simulink model "controller_compare"  (R2023a)
settings: Solver=VariableStepAuto  StartTime=0.0  StopTime=10.0  RelTol=1e-3
model workspace (MAT data in the model file):
  xinit = 1
settings Model: Creator=belov  LastModifiedBy=belov

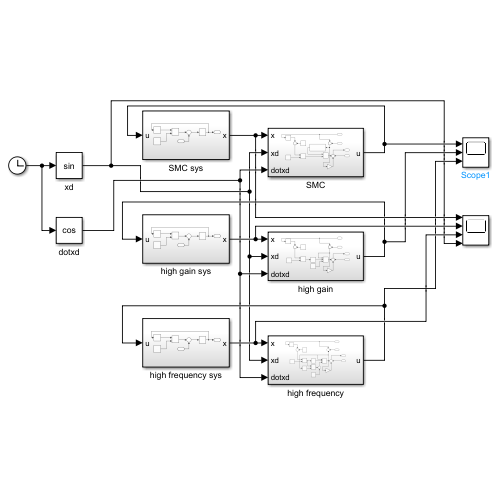
[thumbnail: Simulink's stored preview of the top-level diagram]
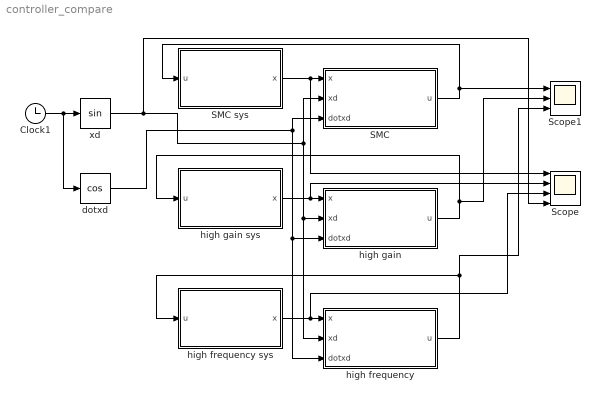
== system controller_compare ==
  Clock1 : Clock
  SMC : Subsystem
  SMC sys : Subsystem
  Scope : Scope  NumInputPorts=4
  Scope1 : Scope  NumInputPorts=3
  dotxd : Trigonometry  Operator=cos
  high frequency : Subsystem
  high frequency sys : Subsystem
  high gain : Subsystem
  high gain sys : Subsystem
  xd : Trigonometry
  wires:
  high frequency sys/1(x) -> Scope/3, high frequency/1(x)
  high gain sys/1(x) -> Scope/2, high gain/1(x)
  SMC sys/1(x) -> Scope/1, SMC/1(x)
  SMC/1(u) -> Scope1/1, SMC sys/1(u)
  high gain/1(u) -> Scope1/2, high gain sys/1(u)
  high frequency/1(u) -> Scope1/3, high frequency sys/1(u)
  xd/1 -> Scope/4, high frequency/2(xd), high gain/2(xd), SMC/2(xd)
  dotxd/1 -> SMC/3(dotxd), high frequency/3(dotxd), high gain/3(dotxd)
  Clock1/1 -> dotxd/1, xd/1

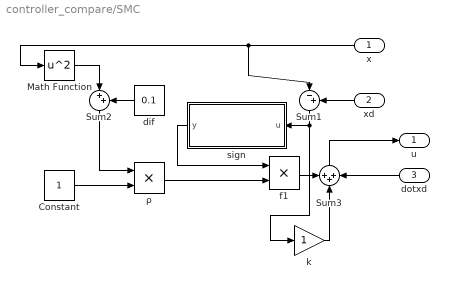
== system controller_compare/SMC ==
  x : Inport
  xd : Inport  Port=2
  dotxd : Inport  Port=3
  Constant : Constant
  Math Function : Math  Operator=square
  Sum1 : Sum  Inputs=|-+
  Sum2 : Sum  Inputs=|++
  Sum3 : Sum  Inputs=+++
  dif : Constant  Value=0.1
  f1 : Product  Inputs=**
  k : Gain
  sign : MATLAB Function  TreatAsAtomicUnit=on
  ρ : Product  Inputs=**
  u : Outport
  wires:
  Math Function/1 -> Sum2/1
  dotxd/1 -> Sum3/3
  xd/1 -> Sum1/2
  x/1 -> Sum1/1, Math Function/1
  Sum1/1 -> k/1, sign/1(u)
  Constant/1 -> ρ/2
  k/1 -> Sum3/2
  Sum2/1 -> ρ/1
  f1/1 -> Sum3/1
  dif/1 -> Sum2/2
  Sum3/1 -> u/1
  ρ/1 -> f1/2
  sign/1(y) -> f1/1

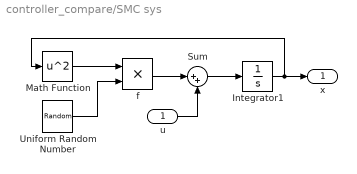
== system controller_compare/SMC sys ==
  u : Inport
  Integrator1 : Integrator  InitialCondition=1
  Math Function : Math  Operator=square
  Sum : Sum  Inputs=|++
  Uniform Random Number : UniformRandomNumber  SampleTime=0.1
  f : Product  Inputs=**
  x : Outport
  wires:
  Math Function/1 -> f/1
  f/1 -> Sum/1
  u/1 -> Sum/2
  Uniform Random Number/1 -> f/2
  Integrator1/1 -> Math Function/1, x/1
  Sum/1 -> Integrator1/1

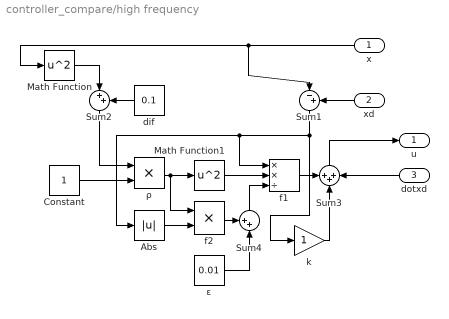
== system controller_compare/high frequency ==
  x : Inport
  xd : Inport  Port=2
  dotxd : Inport  Port=3
  Abs : Abs  SaturateOnIntegerOverflow=off
  Constant : Constant
  Math Function : Math  Operator=square
  Math Function1 : Math  Operator=square
  Sum1 : Sum  Inputs=|-+
  Sum2 : Sum  Inputs=|++
  Sum3 : Sum  Inputs=+++
  Sum4 : Sum  Inputs=++|
  dif : Constant  Value=0.1
  f1 : Product  Inputs=**/
  f2 : Product  Inputs=**
  k : Gain
  ε : Constant  Value=0.01
  ρ : Product  Inputs=**
  u : Outport
  wires:
  Math Function/1 -> Sum2/1
  dotxd/1 -> Sum3/3
  xd/1 -> Sum1/2
  x/1 -> Sum1/1, Math Function/1
  Sum1/1 -> k/1, f1/1, Abs/1
  Constant/1 -> ρ/2
  ρ/1 -> f2/1, Math Function1/1
  k/1 -> Sum3/2
  Sum2/1 -> ρ/1
  f1/1 -> Sum3/1
  dif/1 -> Sum2/2
  Sum3/1 -> u/1
  Math Function1/1 -> f1/2
  Abs/1 -> f2/2
  Sum4/1 -> f1/3
  f2/1 -> Sum4/1
  ε/1 -> Sum4/2

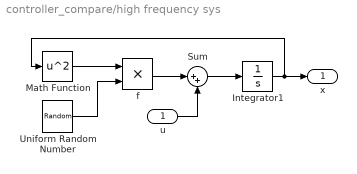
== system controller_compare/high frequency sys ==
  u : Inport
  Integrator1 : Integrator  InitialCondition=1
  Math Function : Math  Operator=square
  Sum : Sum  Inputs=|++
  Uniform Random Number : UniformRandomNumber  SampleTime=0.1
  f : Product  Inputs=**
  x : Outport
  wires:
  Math Function/1 -> f/1
  f/1 -> Sum/1
  u/1 -> Sum/2
  Uniform Random Number/1 -> f/2
  Integrator1/1 -> Math Function/1, x/1
  Sum/1 -> Integrator1/1

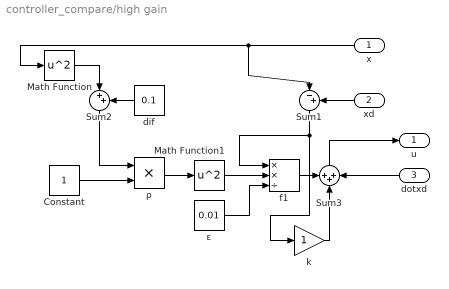
== system controller_compare/high gain ==
  x : Inport
  xd : Inport  Port=2
  dotxd : Inport  Port=3
  Constant : Constant
  Math Function : Math  Operator=square
  Math Function1 : Math  Operator=square
  Sum1 : Sum  Inputs=|-+
  Sum2 : Sum  Inputs=|++
  Sum3 : Sum  Inputs=+++
  dif : Constant  Value=0.1
  f1 : Product  Inputs=**/
  k : Gain
  ε : Constant  Value=0.01
  ρ : Product  Inputs=**
  u : Outport
  wires:
  ε/1 -> f1/3
  Math Function1/1 -> f1/2
  Sum3/1 -> u/1
  dif/1 -> Sum2/2
  f1/1 -> Sum3/1
  Sum2/1 -> ρ/1
  k/1 -> Sum3/2
  ρ/1 -> Math Function1/1
  Constant/1 -> ρ/2
  Sum1/1 -> f1/1, k/1
  x/1 -> Math Function/1, Sum1/1
  xd/1 -> Sum1/2
  dotxd/1 -> Sum3/3
  Math Function/1 -> Sum2/1

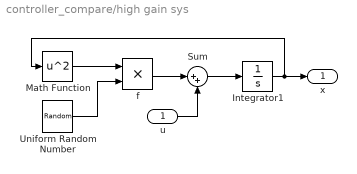
== system controller_compare/high gain sys ==
  u : Inport
  Integrator1 : Integrator  InitialCondition=1
  Math Function : Math  Operator=square
  Sum : Sum  Inputs=|++
  Uniform Random Number : UniformRandomNumber  SampleTime=0.1
  f : Product  Inputs=**
  x : Outport
  wires:
  Sum/1 -> Integrator1/1
  Integrator1/1 -> x/1, Math Function/1
  Uniform Random Number/1 -> f/2
  u/1 -> Sum/2
  f/1 -> Sum/1
  Math Function/1 -> f/1

== matlab function controller_compare/SMC/sign ==
  data: u input; y output
function y = signfunc(u)

y = sign(u);
